simulink model "BBB_Gyro_Test"  (R2013a)
settings: Solver=FixedStepDiscrete  StartTime=0.0  StopTime=inf  FixedStep=0.01  RelTol=1e-3
settings Model: SimulationMode=external  ExtModeTrigDuration=100  Creator=rdustinkahawita  LastModifiedBy=rdustinkahawita
settings OptimizationCC: OptimizeModelRefInitCode=on  LifeSpan=1
settings DebuggingCC: SolverPrmCheckMsg=none  StrictBusMsg=Warning
settings HardwareCC: ProdLargestAtomicInteger=Long  ProdLargestAtomicFloat=Double  ProdEndianess=LittleEndian  ProdHWDeviceType=ARM Compatible->ARM Cortex
settings RTWCC: SystemTargetFile=realtime.tlc  GenerateMakefile=off  TemplateMakefile=realtime.tmf  Description=Run on Target Hardware  RTWVerbose=off  ProcessScript=realtime_make_rtw_hook
settings STFCustomTargetCC: TargetLibSuffix=.a  GenerateSampleERTMain=on  ERTCustomFileBanners=on  SupportNonInlinedSFcns=off  SupportVariableSizeSignals=on  MATLABClassNameForMDSCustomization=Simulink.SoftwareTarget.ERTCustomization  SystemTargetFile=realtime.tlc
settings ERTTargetCC: ParMdlRefBuildCompliant=off  CompOptLevelCompliant=off  ConcurrentExecutionCompliant=off  CombineOutputUpdateFcns=off  ERTFirstTimeCompliant=off  SupportContinuousTime=on  SupportVariableSizeSignals=on  ModelStepFunctionPrototypeControlCompliant=off  CPPClassGenCompliant=off  ExtMode=on  ExtModeMexArgs='192.168.7.2' 0 17725  ERTSrcFileBannerTemplate=realtime_code_template.cgt  ERTHdrFileBannerTemplate=realtime_code_template.cgt  ERTDataSrcFileTemplate=realtime_code_template.cgt  ERTDataHdrFileTemplate=realtime_code_template.cgt  ERTCustomFileTemplate=realtime_file_process.tlc

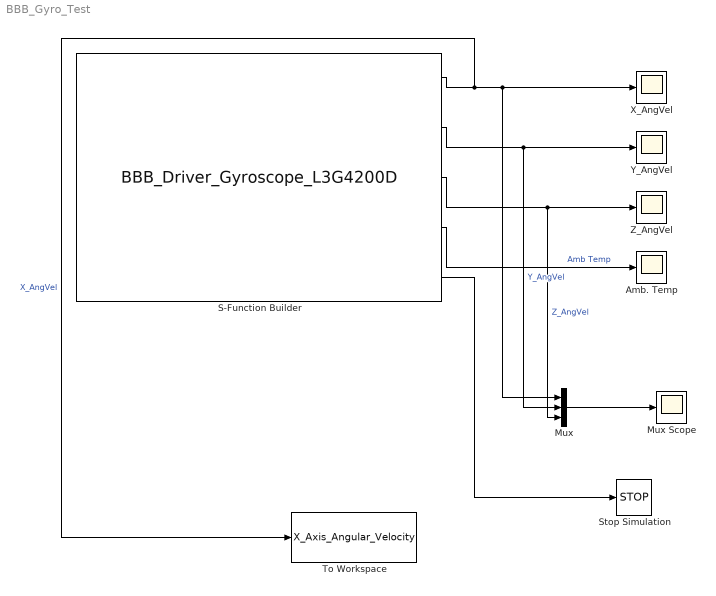
== system BBB_Gyro_Test ==
  Amb. Temp : Scope
      settings: YMin=15.2  YMax=16.8  SaveName=ScopeData3
  Mux : Mux  Inputs=3
  Mux Scope : Scope
      settings: ShowLegends=on  TimeRange=20  YMin=-150  YMax=175  SaveName=ScopeData4
  S-Function Builder : S-Function  InitFcn=try, set_param(gcb,'FunctionName','BBB_Driver_Gyroscope_L3G4200D'), end  FunctionName=BBB_Driver_Gyroscope_L3G4200D  Parameters=uint8(1),uint8(104),uint8(1),uint8(1)  SFunctionModules=BBB_Driver_Gyroscope_L3G4200D_wrapper  EnableBusSupport=off
      mask init:
      | val = [[.9  0.75 0.75 1 1 .9 .9 1]',[1 1 0.75 0.75 .9 .9 1 .9]'];try , sys = get_param(gcb,'SfunBuilderFcnName');if isempty(sys), sys = get_param(gcb,'FunctionName'); end,catch, sys = get_param(gcb,'FunctionName'); end
      settings: CopyFcn=set_param(gcbh,'LinkStatus','none')  PreSaveFcn=try, set_param(gcb,'FunctionName','BBB_Driver_Gyroscope_L3G4200D'), end  OpenFcn=sfunctionwizard(gcbh)
      mask Display: plot(val(:,1),val(:,2)),disp(sys), port_label('output',1,'outAngVel_X'), port_label('output',2,'outAngVel_Y'), port_label('output',3,'outAngVel_Z'), port_label('output',4,'outAmbTemp'), port_label('output',5,'outSimStop')
  Stop Simulation : Stop
  To Workspace : ToWorkspace  VariableName=X_Axis_Angular_Velocity  SampleTime=-1
  X_AngVel : Scope
      settings: TimeRange=10  YMin=-300  YMax=250
  Y_AngVel : Scope
      settings: YMin=-300  YMax=300
  Z_AngVel : Scope
      settings: YMin=-300  YMax=250  SaveName=ScopeData2
  wires:
  S-Function Builder/1 -> To Workspace/1, X_AngVel/1, Mux/1  "X_AngVel"
  S-Function Builder/2 -> Y_AngVel/1, Mux/2  "Y_AngVel"
  S-Function Builder/3 -> Mux/3, Z_AngVel/1  "Z_AngVel"
  S-Function Builder/4 -> Amb. Temp/1  "Amb Temp"
  Mux/1 -> Mux Scope/1
  S-Function Builder/5 -> Stop Simulation/1
